simulink model "ad9361_sim"  (R2016b)
settings: Solver=ode45  StartTime=0.0  StopTime=Inf  RelTol=1e-3  EnableMultiTasking=on
libraries: dspsrcs4 x2, simulink x2
settings Model: Creator=ACozma  LastModifiedBy=DPu1
settings DataIOCC: LimitDataPoints=on  SaveFormat=Array
settings OptimizationCC: LifeSpan=inf
settings DebuggingCC: UnderspecifiedInitializationDetection=Classic  MergeDetectMultiDrivingBlocksExec=none  SolverPrmCheckMsg=warning  SFUnexpectedBacktrackingDiag=warning  SFNoUnconditionalDefaultTransitionDiag=warning  SFExecutionAtInitializationDiag=none
settings HardwareCC: ProdBitPerPointer=32  ProdBitPerSizeT=32  ProdBitPerPtrDiffT=32  ProdLargestAtomicFloat=None  ProdIntDivRoundTo=Undefined  ProdEndianess=Unspecified  ProdWordSize=32  ProdHWDeviceType=32-bit Generic
settings ModelReferenceCC: PropagateSignalLabelsOutOfModel=off
settings GRTTargetCC: TargetLangStandard=C89/C90 (ANSI)  GeneratePreprocessorConditionals=Disable all
settings ConfigComp: CovMetricSettings=dw  CovHtmlReporting=on  CovSaveCumulativeToWorkspaceVar=on  CovSaveSingleToWorkspaceVar=on  CovExternalEMLEnable=off  CovSFcnEnable=off

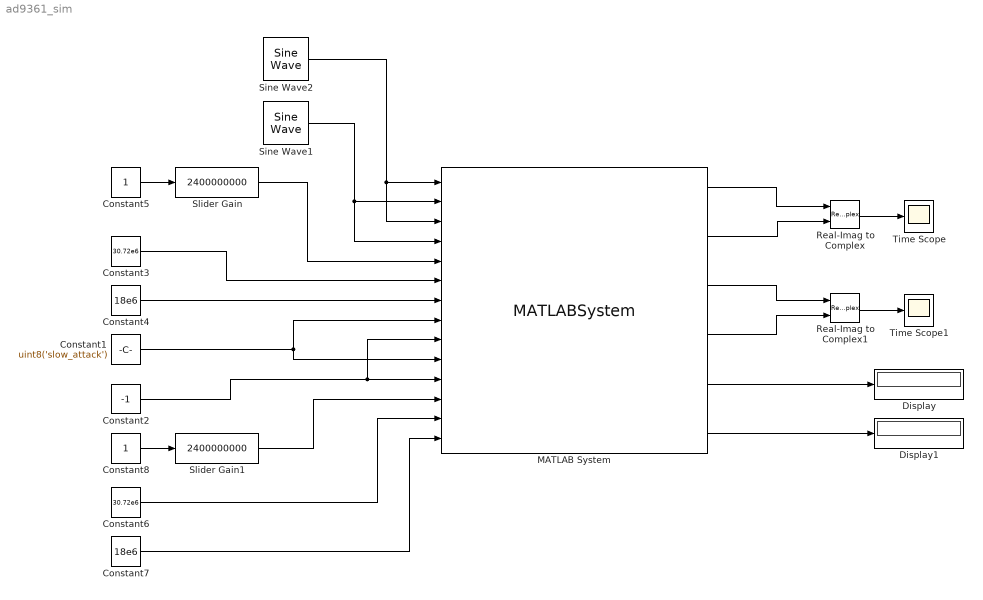
== system ad9361_sim ==
  Constant1 : Constant  Value=uint8('slow_attack')  SampleTime=-1
  Constant2 : Constant  Value=-1  SampleTime=-1
  Constant3 : Constant  Value=30.72e6  SampleTime=-1
  Constant4 : Constant  Value=18e6  SampleTime=-1
  Constant5 : Constant  SampleTime=-1
  Constant6 : Constant  Value=30.72e6  SampleTime=-1
  Constant7 : Constant  Value=18e6  SampleTime=-1
  Constant8 : Constant  SampleTime=-1
  Display : Display
  Display1 : Display
  MATLAB System : MATLABSystem  DialogController=sysobjdialog.BlockDynDialog  System=iio_sys_obj  ip_address=192.168.3.2  dev_name=ad9361  in_ch_no=4  in_ch_size=32768  out_ch_no=4  out_ch_size=8192  SimulateUsing=Interpreted execution
      mask Type: iio_sys_obj
      mask Display:
      | disp('ad9361');
      | port_label('input',1,'DATA_IN1');
      | port_label('input',2,'DATA_IN2');
      | port_label('input',3,'DATA_IN3');
      | port_label('input',4,'DATA_IN4');
      | port_label('input',5,'RX_LO_FREQ');
      | port_label('input',6,'RX_SAMPLING_FREQ');
      | port_label('input',7,'RX_RF_BANDWIDTH');
      | port_label('input',8,'RX1_GAIN_MODE');
      | port_label('input',9,'RX1_GAIN');
      | port_label('input',10,'RX2_GAIN_MODE');
      | port_label('input',11,'RX2_GAIN');
      | port_label('input',12,'TX_LO_FREQ');
      | port_label('input',13,'TX_SAMPLING_FREQ');
      | port_label('input',14,'TX_RF_BANDWIDTH');
      | port_label('output',1,'DATA_OUT1');
      | port_label('output',2,'DATA_OUT2');
      | port_label('output',3,'DATA_OUT3');
      | port_label('output',4,'DATA_OUT4');
      | port_label('output',5,'RX1_RSSI');
      | port_label('output',6,'RX2_RSSI');
  Real-Imag to Complex : RealImagToComplex
  Real-Imag to Complex1 : RealImagToComplex
  Sine Wave1 : dspsrcs4/Sine Wave  Amplitude=32768  Frequency=100  Phase=pi/2  SampleMode=Discrete  OutComplex=Real  CompMethod=Trigonometric fcn  TableSize=Speed  SampleTime=1/10000  SamplesPerFrame=32768  ResetState=Catch up to simulation time  OutputFrames=on  dataType=double  wordLen=16  udDataType=sfix(16)  fracBitsMode=Best precision  numFracBits=15  OutDataTypeStr=double  LastOutDataTypeStr=double
  Sine Wave2 : dspsrcs4/Sine Wave  Amplitude=32768  Frequency=100  Phase=0  SampleMode=Discrete  OutComplex=Real  CompMethod=Trigonometric fcn  TableSize=Speed  SampleTime=1/10000  SamplesPerFrame=32768  ResetState=Catch up to simulation time  OutputFrames=on  dataType=double  wordLen=16  udDataType=sfix(16)  fracBitsMode=Best precision  numFracBits=15  OutDataTypeStr=double  LastOutDataTypeStr=double
  Slider Gain : simulink/Math Operations/Slider Gain  low=200000  gain=2400000000  high=6000000000
  Slider Gain1 : simulink/Math Operations/Slider Gain  low=200000  gain=2400000000  high=6000000000
  Time Scope : Scope
  Time Scope1 : Scope
  wires:
  Constant5/1 -> Slider Gain/1
  Constant8/1 -> Slider Gain1/1
  MATLAB System/1 -> Real-Imag to Complex/1
  MATLAB System/2 -> Real-Imag to Complex/2
  Sine Wave2/1 -> MATLAB System/1, MATLAB System/3
  Sine Wave1/1 -> MATLAB System/4, MATLAB System/2
  Real-Imag to Complex/1 -> Time Scope/1
  MATLAB System/5 -> Display/1
  MATLAB System/6 -> Display1/1
  Real-Imag to Complex1/1 -> Time Scope1/1
  MATLAB System/3 -> Real-Imag to Complex1/1
  MATLAB System/4 -> Real-Imag to Complex1/2
  Slider Gain/1 -> MATLAB System/5
  Constant3/1 -> MATLAB System/6
  Constant4/1 -> MATLAB System/7
  Constant1/1 -> MATLAB System/8, MATLAB System/10
  Constant2/1 -> MATLAB System/11, MATLAB System/9
  Slider Gain1/1 -> MATLAB System/12
  Constant6/1 -> MATLAB System/13
  Constant7/1 -> MATLAB System/14
